simulink model "Prp_TrqDesCoord"  (R2018a)
settings: configuration reference "cs_ert" (kept outside this file)
settings Model: DataDictionary=Prp_TrqDesCoord.sldd  Creator=zhoutinglin  LastModifiedBy=zhoutinglin

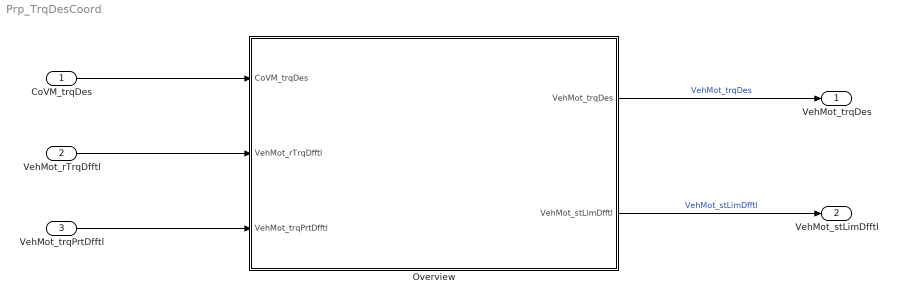
== system Prp_TrqDesCoord ==
  CoVM_trqDes : Inport  Description=Propulsion torque order after ESP-torque intervention coordination (wheel torque)  OutMin=-3000  OutMax=3000  OutDataTypeStr=Torq  Unit=Nm  PortDimensions=[1 1]
  VehMot_rTrqDfftl : Inport  Description=Torque ratio of differential  Port=2  OutMin=-100  OutMax=100  OutDataTypeStr=Ratio_100  PortDimensions=[1 1]
  VehMot_trqPrtDfftl : Inport  Description=Differential protection torque  Port=3  OutMin=-3000  OutMax=3000  OutDataTypeStr=Torq  Unit=Nm  PortDimensions=[1 1]
  Overview : Subsystem
  VehMot_trqDes : Outport
  VehMot_stLimDfftl : Outport  Port=2
  wires:
  CoVM_trqDes/1 -> Overview/1(CoVM_trqDes)
  VehMot_rTrqDfftl/1 -> Overview/2(VehMot_rTrqDfftl)
  VehMot_trqPrtDfftl/1 -> Overview/3(VehMot_trqPrtDfftl)
  Overview/1(VehMot_trqDes) -> VehMot_trqDes/1  "VehMot_trqDes"
  Overview/2(VehMot_stLimDfftl) -> VehMot_stLimDfftl/1  "VehMot_stLimDfftl"

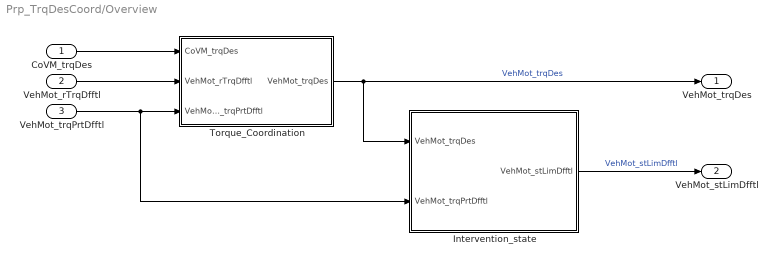
== system Prp_TrqDesCoord/Overview ==
  CoVM_trqDes : Inport  Tag=Nm
  VehMot_rTrqDfftl : Inport  Port=2
  VehMot_trqPrtDfftl : Inport  Tag=Nm  Port=3
  Intervention_state : Subsystem
  Torque_Coordination : Subsystem
  VehMot_trqDes : Outport  Tag=Nm
  VehMot_stLimDfftl : Outport  Port=2
  wires:
  Intervention_state/1(VehMot_stLimDfftl) -> VehMot_stLimDfftl/1  "VehMot_stLimDfftl"
  VehMot_rTrqDfftl/1 -> Torque_Coordination/2(VehMot_rTrqDfftl)
  CoVM_trqDes/1 -> Torque_Coordination/1(CoVM_trqDes)
  VehMot_trqPrtDfftl/1 -> Intervention_state/2(VehMot_trqPrtDfftl), Torque_Coordination/3(VehMot_trqPrtDfftl)
  Torque_Coordination/1(VehMot_trqDes) -> VehMot_trqDes/1, Intervention_state/1(VehMot_trqDes)  "VehMot_trqDes"

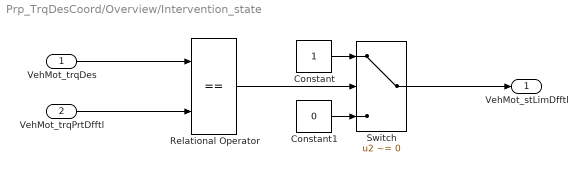
== system Prp_TrqDesCoord/Overview/Intervention_state ==
  VehMot_trqDes : Inport
  VehMot_trqPrtDfftl : Inport  Port=2
  Constant : Constant  OutDataTypeStr=Inherit: Inherit via back propagation
  Constant1 : Constant  Value=0  OutDataTypeStr=Inherit: Inherit via back propagation
  Relational Operator : RelationalOperator  Operator===  OutDataTypeStr=boolean  RndMeth=Simplest  InputSameDT=on
  Switch : Switch  Criteria=u2 ~= 0  InputSameDT=on
  VehMot_stLimDfftl : Outport
  wires:
  Switch/1 -> VehMot_stLimDfftl/1
  Constant1/1 -> Switch/3
  Constant/1 -> Switch/1
  Relational Operator/1 -> Switch/2
  VehMot_trqPrtDfftl/1 -> Relational Operator/2
  VehMot_trqDes/1 -> Relational Operator/1

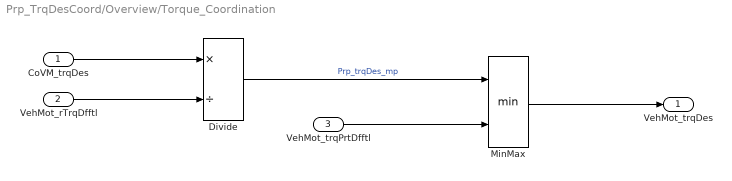
== system Prp_TrqDesCoord/Overview/Torque_Coordination ==
  CoVM_trqDes : Inport  Tag=Nm
  VehMot_rTrqDfftl : Inport  Tag=-  Port=2
  VehMot_trqPrtDfftl : Inport  Tag=Nm  Port=3
  Divide : Product  Inputs=*/  OutDataTypeStr=Inherit: Inherit via back propagation
  MinMax : MinMax  Inputs=2  InputSameDT=on
  VehMot_trqDes : Outport
  wires:
  VehMot_trqPrtDfftl/1 -> MinMax/2
  CoVM_trqDes/1 -> Divide/1
  Divide/1 -> MinMax/1  "Prp_trqDes_mp"
  VehMot_rTrqDfftl/1 -> Divide/2
  MinMax/1 -> VehMot_trqDes/1
